simulink model "cardio"  (Simulink 7.2)
settings: Solver=ode45  StartTime=0.0  StopTime=10.0  RelTol=1e-3
undefined symbols (not defined in the file): ln
(part 2 of 2)

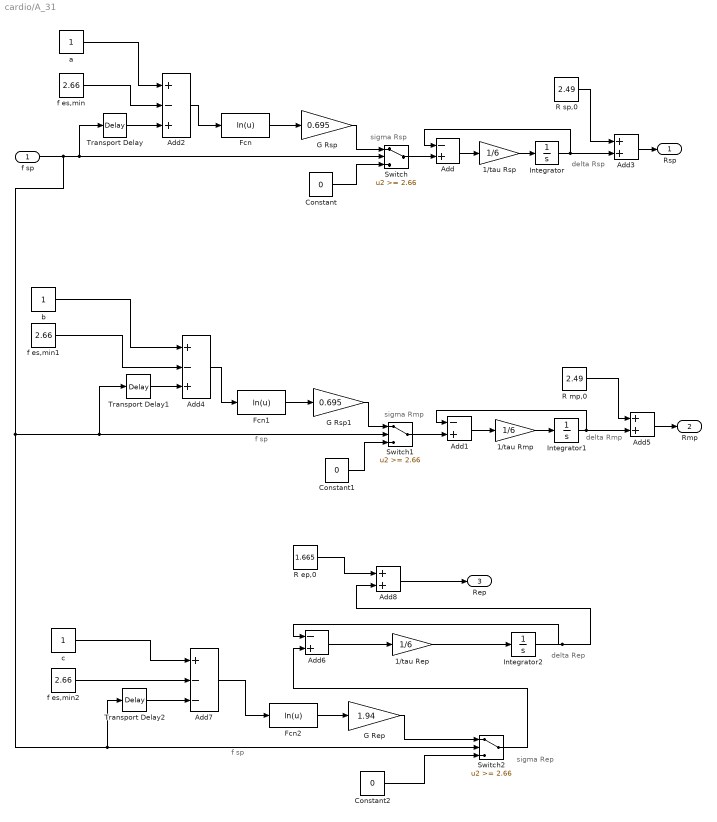
== system cardio/A_31 ==
  note: sigma Rep
  note: delta Rep
  note: f sp
  note: f sp
  note: delta Rmp
  note: sigma Rmp
  note: delta Rsp
  note: sigma Rsp
  f sp : Inport  OutDataType=sfix(16)  OutScaling=2^0
  1/tau Rep : Gain  Gain=1/6  ParameterDataType=sfix(16)  ParameterScaling=2^0  OutDataType=sfix(16)  OutScaling=2^0
  1/tau Rmp : Gain  Gain=1/6  ParameterDataType=sfix(16)  ParameterScaling=2^0  OutDataType=sfix(16)  OutScaling=2^0
  1/tau Rsp : Gain  Gain=1/6  ParameterDataType=sfix(16)  ParameterScaling=2^0  OutDataType=sfix(16)  OutScaling=2^0
  Add : Sum  Inputs=-+  OutDataType=sfix(16)  OutScaling=2^-10
  Add1 : Sum  Inputs=-+  OutDataType=sfix(16)  OutScaling=2^-10
  Add2 : Sum  Inputs=+-+  OutDataType=sfix(16)  OutScaling=2^-10
  Add3 : Sum  OutDataType=sfix(16)  OutScaling=2^-10
  Add4 : Sum  Inputs=+-+  OutDataType=sfix(16)  OutScaling=2^-10
  Add5 : Sum  OutDataType=sfix(16)  OutScaling=2^-10
  Add6 : Sum  Inputs=-+  OutDataType=sfix(16)  OutScaling=2^-10
  Add7 : Sum  Inputs=+--  OutDataType=sfix(16)  OutScaling=2^-10
  Add8 : Sum  OutDataType=sfix(16)  OutScaling=2^-10
  Constant : Constant  Value=0  OutDataType=sfix(16)  OutScaling=2^0
  Constant1 : Constant  Value=0  OutDataType=sfix(16)  OutScaling=2^0
  Constant2 : Constant  Value=0  OutDataType=sfix(16)  OutScaling=2^0
  Fcn : Fcn  Expr=ln(u)
  Fcn1 : Fcn  Expr=ln(u)
  Fcn2 : Fcn  Expr=ln(u)
  G Rep : Gain  Gain=1.94  ParameterDataType=sfix(16)  ParameterScaling=2^0  OutDataType=sfix(16)  OutScaling=2^0
  G Rsp : Gain  Gain=0.695  ParameterDataType=sfix(16)  ParameterScaling=2^0  OutDataType=sfix(16)  OutScaling=2^0
  G Rsp1 : Gain  Gain=0.695  ParameterDataType=sfix(16)  ParameterScaling=2^0  OutDataType=sfix(16)  OutScaling=2^0
  Integrator : Integrator
  Integrator1 : Integrator
  Integrator2 : Integrator
  R ep,0 : Constant  Value=1.665  OutDataType=sfix(16)  OutScaling=2^0
  R mp,0 : Constant  Value=2.49  OutDataType=sfix(16)  OutScaling=2^0
  R sp,0 : Constant  Value=2.49  OutDataType=sfix(16)  OutScaling=2^0
  Switch : Switch  Threshold=2.66  OutDataType=sfix(16)  OutScaling=2^0
  Switch1 : Switch  Threshold=2.66  OutDataType=sfix(16)  OutScaling=2^0
  Switch2 : Switch  Threshold=2.66  OutDataType=sfix(16)  OutScaling=2^0
  Transport Delay : TransportDelay  DelayTime=2
  Transport Delay1 : TransportDelay  DelayTime=2
  Transport Delay2 : TransportDelay  DelayTime=2
  a : Constant  OutDataType=sfix(16)  OutScaling=2^0
  b : Constant  OutDataType=sfix(16)  OutScaling=2^0
  c : Constant  OutDataType=sfix(16)  OutScaling=2^0
  f es,min : Constant  Value=2.66  OutDataType=sfix(16)  OutScaling=2^0
  f es,min1 : Constant  Value=2.66  OutDataType=sfix(16)  OutScaling=2^0
  f es,min2 : Constant  Value=2.66  OutDataType=sfix(16)  OutScaling=2^0
  Rsp : Outport  OutDataType=sfix(16)  OutScaling=2^0
  Rmp : Outport  Port=2  OutDataType=sfix(16)  OutScaling=2^0
  Rep : Outport  Port=3  OutDataType=sfix(16)  OutScaling=2^0
  wires:
  Add4/1 -> Fcn1/1
  Switch1/1 -> Add1/2
  Constant1/1 -> Switch1/3
  R mp,0/1 -> Add5/1
  Add5/1 -> Rmp/1
  f es,min/1 -> Add2/2
  a/1 -> Add2/1
  Constant/1 -> Switch/3
  Switch/1 -> Add/2
  R sp,0/1 -> Add3/1
  Transport Delay/1 -> Add2/3
  Transport Delay2/1 -> Add7/3
  R ep,0/1 -> Add8/1
  Add8/1 -> Rep/1
  f es,min2/1 -> Add7/2
  c/1 -> Add7/1
  Add7/1 -> Fcn2/1
  Fcn2/1 -> G Rep/1
  G Rep/1 -> Switch2/1
  Constant2/1 -> Switch2/3
  Switch2/1 -> Add6/2
  Integrator2/1 -> Add8/2, Add6/1
  Add6/1 -> 1/tau Rep/1
  1/tau Rep/1 -> Integrator2/1
  Transport Delay1/1 -> Add4/3
  f es,min1/1 -> Add4/2
  b/1 -> Add4/1
  Fcn1/1 -> G Rsp1/1
  G Rsp1/1 -> Switch1/1
  Integrator1/1 -> Add5/2, Add1/1
  Add1/1 -> 1/tau Rmp/1
  1/tau Rmp/1 -> Integrator1/1
  Add3/1 -> Rsp/1
  Add2/1 -> Fcn/1
  Fcn/1 -> G Rsp/1
  G Rsp/1 -> Switch/1
  f sp/1 -> Transport Delay2/1, Switch2/2, Transport Delay1/1, Switch1/2, Switch/2, Transport Delay/1
  Integrator/1 -> Add3/2, Add/1
  Add/1 -> 1/tau Rsp/1
  1/tau Rsp/1 -> Integrator/1

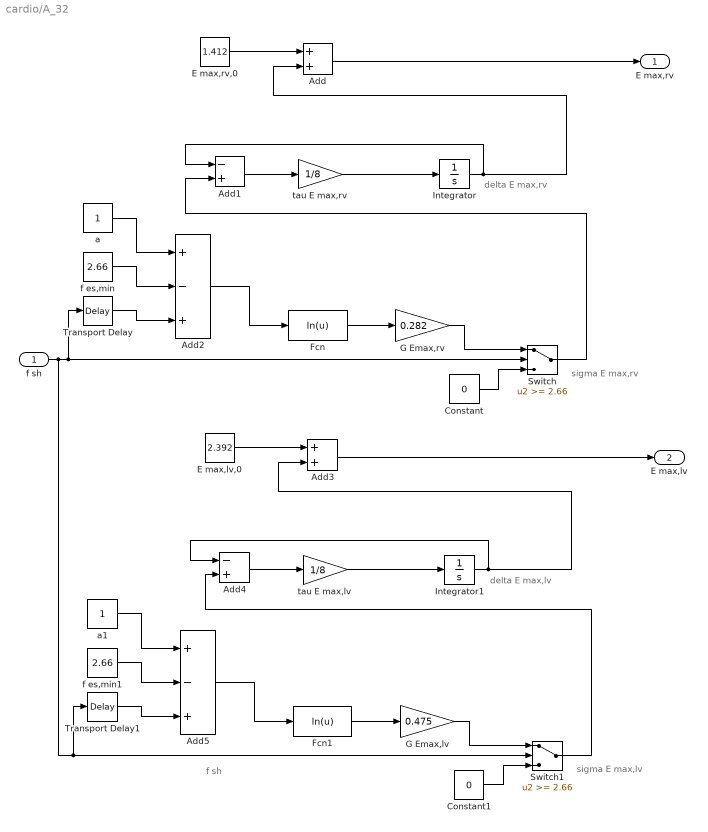
== system cardio/A_32 ==
  note: f sh
  note: sigma E max,lv
  note: delta E max,lv
  note: sigma E max,rv
  note: delta E max,rv
  f sh : Inport  OutDataType=sfix(16)  OutScaling=2^0
  Add : Sum  OutDataType=sfix(16)  OutScaling=2^-10
  Add1 : Sum  Inputs=-+  OutDataType=sfix(16)  OutScaling=2^-10
  Add2 : Sum  Inputs=+-+  OutDataType=sfix(16)  OutScaling=2^-10
  Add3 : Sum  OutDataType=sfix(16)  OutScaling=2^-10
  Add4 : Sum  Inputs=-+  OutDataType=sfix(16)  OutScaling=2^-10
  Add5 : Sum  Inputs=+-+  OutDataType=sfix(16)  OutScaling=2^-10
  Constant : Constant  Value=0  OutDataType=sfix(16)  OutScaling=2^0
  Constant1 : Constant  Value=0  OutDataType=sfix(16)  OutScaling=2^0
  E max,lv,0 : Constant  Value=2.392  OutDataType=sfix(16)  OutScaling=2^0
  E max,rv,0 : Constant  Value=1.412  OutDataType=sfix(16)  OutScaling=2^0
  Fcn : Fcn  Expr=ln(u)
  Fcn1 : Fcn  Expr=ln(u)
  G Emax,lv : Gain  Gain=0.475  ParameterDataType=sfix(16)  ParameterScaling=2^0  OutDataType=sfix(16)  OutScaling=2^0
  G Emax,rv : Gain  Gain=0.282  ParameterDataType=sfix(16)  ParameterScaling=2^0  OutDataType=sfix(16)  OutScaling=2^0
  Integrator : Integrator
  Integrator1 : Integrator
  Switch : Switch  Threshold=2.66  OutDataType=sfix(16)  OutScaling=2^0
  Switch1 : Switch  Threshold=2.66  OutDataType=sfix(16)  OutScaling=2^0
  Transport Delay : TransportDelay  DelayTime=2
  Transport Delay1 : TransportDelay  DelayTime=2
  a : Constant  OutDataType=sfix(16)  OutScaling=2^0
  a1 : Constant  OutDataType=sfix(16)  OutScaling=2^0
  f es,min : Constant  Value=2.66  OutDataType=sfix(16)  OutScaling=2^0
  f es,min1 : Constant  Value=2.66  OutDataType=sfix(16)  OutScaling=2^0
  tau E max,lv : Gain  Gain=1/8  ParameterDataType=sfix(16)  ParameterScaling=2^0  OutDataType=sfix(16)  OutScaling=2^0
  tau E max,rv : Gain  Gain=1/8  ParameterDataType=sfix(16)  ParameterScaling=2^0  OutDataType=sfix(16)  OutScaling=2^0
  E max,rv : Outport  OutDataType=sfix(16)  OutScaling=2^0
  E max,lv : Outport  Port=2  OutDataType=sfix(16)  OutScaling=2^0
  wires:
  a1/1 -> Add5/1
  f es,min1/1 -> Add5/2
  Transport Delay1/1 -> Add5/3
  Add5/1 -> Fcn1/1
  G Emax,lv/1 -> Switch1/1
  Fcn1/1 -> G Emax,lv/1
  Constant1/1 -> Switch1/3
  Switch1/1 -> Add4/2
  Add4/1 -> tau E max,lv/1
  tau E max,lv/1 -> Integrator1/1
  Integrator1/1 -> Add3/2, Add4/1
  E max,lv,0/1 -> Add3/1
  Add3/1 -> E max,lv/1
  a/1 -> Add2/1
  f es,min/1 -> Add2/2
  Transport Delay/1 -> Add2/3
  Add2/1 -> Fcn/1
  G Emax,rv/1 -> Switch/1
  Fcn/1 -> G Emax,rv/1
  Constant/1 -> Switch/3
  f sh/1 -> Transport Delay1/1, Switch1/2, Transport Delay/1, Switch/2
  Switch/1 -> Add1/2
  Add1/1 -> tau E max,rv/1
  tau E max,rv/1 -> Integrator/1
  Integrator/1 -> Add/2, Add1/1
  E max,rv,0/1 -> Add/1
  Add/1 -> E max,rv/1
